simulink model "Ex3EMT"  (R2023b)
settings: Solver=VariableStepAuto  StartTime=0.0  StopTime=10.0  RelTol=1e-3
undefined symbols (not defined in the file): designMultirateFIR
libraries: dspmlti4 x8, dspstat3 x4
settings Model: Creator=Fartash  LastModifiedBy=Fartash

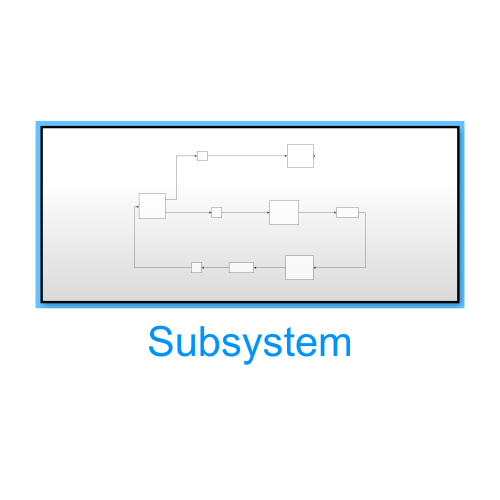
[thumbnail: Simulink's stored preview of the top-level diagram]
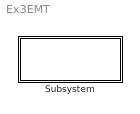
== system Ex3EMT ==
  Subsystem : Subsystem

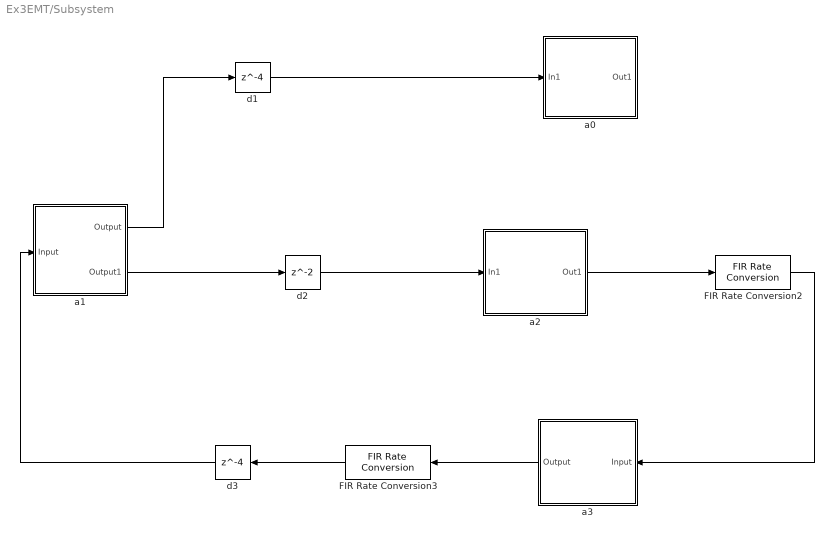
== system Ex3EMT/Subsystem ==
  FIR Rate Conversion2 : dspmlti4/FIR Rate Conversion  FilterSource=Auto  L=1  h=designMultirateFIR(3,2)  M=4  FilterObject=FRC  rateMode=Enforce single-rate processing  AllowArbitraryInputLength=off  roundingMode=Floor  overflowMode=off  firstCoeffDataTypeStr=Inherit: Same word length as input  firstCoeffMin=[]  firstCoeffMax=[]  firstCoeffLastDataTypeStr=Inherit: Same word length as input  outputDataTypeStr=Inherit: Same as accumulator  outputMin=[]  outputMax=[]  outputLastDataTypeStr=Inherit: Same as accumulator
  FIR Rate Conversion3 : dspmlti4/FIR Rate Conversion  FilterSource=Auto  L=3  h=designMultirateFIR(3,2)  M=1  FilterObject=FRC  rateMode=Enforce single-rate processing  AllowArbitraryInputLength=off  roundingMode=Floor  overflowMode=off  firstCoeffDataTypeStr=Inherit: Same word length as input  firstCoeffMin=[]  firstCoeffMax=[]  firstCoeffLastDataTypeStr=Inherit: Same word length as input  outputDataTypeStr=Inherit: Same as accumulator  outputMin=[]  outputMax=[]  outputLastDataTypeStr=Inherit: Same as accumulator
  a0 : Subsystem
  a1 : Subsystem
  a2 : Subsystem
  a3 : Subsystem
  d1 : Delay  DelayLength=4
  d2 : Delay
  d3 : Delay  DelayLength=4
  wires:
  FIR Rate Conversion3/1 -> d3/1
  a2/1(Out1) -> FIR Rate Conversion2/1
  a3/1(Output) -> FIR Rate Conversion3/1
  a1/1(Output) -> d1/1
  a1/2(Output1) -> d2/1
  d2/1 -> a2/1(In1)
  FIR Rate Conversion2/1 -> a3/1(Input)
  d1/1 -> a0/1(In1)
  d3/1 -> a1/1(Input)

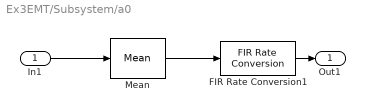
== system Ex3EMT/Subsystem/a0 ==
  In1 : Inport
  FIR Rate Conversion1 : dspmlti4/FIR Rate Conversion  FilterSource=Auto  L=3  h=designMultirateFIR(3,2)  M=1  FilterObject=FRC  rateMode=Enforce single-rate processing  AllowArbitraryInputLength=off  roundingMode=Floor  overflowMode=off  firstCoeffDataTypeStr=Inherit: Same word length as input  firstCoeffMin=[]  firstCoeffMax=[]  firstCoeffLastDataTypeStr=Inherit: Same word length as input  outputDataTypeStr=Inherit: Same as accumulator  outputMin=[]  outputMax=[]  outputLastDataTypeStr=Inherit: Same as accumulator
  Mean : dspstat3/Mean  run=off  InputProcessing=Columns as channels (frame based)  reset_popup=None  directionMode=Each column  dimension=1  roiEnable=off  roiType=Rectangles  roiPortion=Entire ROI  roiOutput=Individual statistics for each ROI  roiFlag=off  roundingMode=Floor  overflowMode=off  outputDataTypeStr=Inherit: Same as accumulator  outputMin=[]  outputMax=[]  outputLastDataTypeStr=Inherit: Same as accumulator
  Out1 : Outport
  wires:
  In1/1 -> Mean/1
  Mean/1 -> FIR Rate Conversion1/1
  FIR Rate Conversion1/1 -> Out1/1

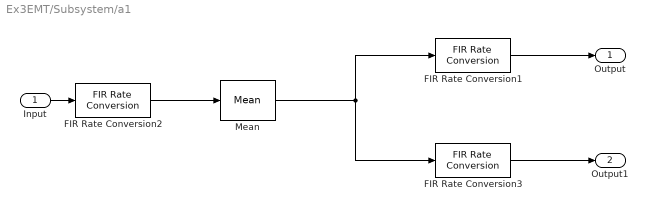
== system Ex3EMT/Subsystem/a1 ==
  Input : Inport
  FIR Rate Conversion1 : dspmlti4/FIR Rate Conversion  FilterSource=Auto  L=2  h=designMultirateFIR(3,2)  M=1  FilterObject=FRC  rateMode=Enforce single-rate processing  AllowArbitraryInputLength=off  roundingMode=Floor  overflowMode=off  firstCoeffDataTypeStr=Inherit: Same word length as input  firstCoeffMin=[]  firstCoeffMax=[]  firstCoeffLastDataTypeStr=Inherit: Same word length as input  outputDataTypeStr=Inherit: Same as accumulator  outputMin=[]  outputMax=[]  outputLastDataTypeStr=Inherit: Same as accumulator
  FIR Rate Conversion2 : dspmlti4/FIR Rate Conversion  FilterSource=Auto  L=4  h=designMultirateFIR(3,2)  M=1  FilterObject=FRC  rateMode=Enforce single-rate processing  AllowArbitraryInputLength=off  roundingMode=Floor  overflowMode=off  firstCoeffDataTypeStr=Inherit: Same word length as input  firstCoeffMin=[]  firstCoeffMax=[]  firstCoeffLastDataTypeStr=Inherit: Same word length as input  outputDataTypeStr=Inherit: Same as accumulator  outputMin=[]  outputMax=[]  outputLastDataTypeStr=Inherit: Same as accumulator
  FIR Rate Conversion3 : dspmlti4/FIR Rate Conversion  FilterSource=Auto  L=1  h=designMultirateFIR(3,2)  M=1  FilterObject=FRC  rateMode=Enforce single-rate processing  AllowArbitraryInputLength=off  roundingMode=Floor  overflowMode=off  firstCoeffDataTypeStr=Inherit: Same word length as input  firstCoeffMin=[]  firstCoeffMax=[]  firstCoeffLastDataTypeStr=Inherit: Same word length as input  outputDataTypeStr=Inherit: Same as accumulator  outputMin=[]  outputMax=[]  outputLastDataTypeStr=Inherit: Same as accumulator
  Mean : dspstat3/Mean  run=off  InputProcessing=Columns as channels (frame based)  reset_popup=None  directionMode=Each column  dimension=1  roiEnable=off  roiType=Rectangles  roiPortion=Entire ROI  roiOutput=Individual statistics for each ROI  roiFlag=off  roundingMode=Floor  overflowMode=off  outputDataTypeStr=Inherit: Same as accumulator  outputMin=[]  outputMax=[]  outputLastDataTypeStr=Inherit: Same as accumulator
  Output : Outport
  Output1 : Outport  Port=2
  wires:
  Input/1 -> FIR Rate Conversion2/1
  FIR Rate Conversion2/1 -> Mean/1
  FIR Rate Conversion3/1 -> Output1/1
  FIR Rate Conversion1/1 -> Output/1
  Mean/1 -> FIR Rate Conversion3/1, FIR Rate Conversion1/1

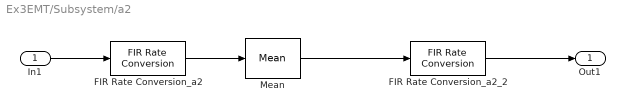
== system Ex3EMT/Subsystem/a2 ==
  In1 : Inport
  FIR Rate Conversion_a2 : dspmlti4/FIR Rate Conversion  FilterSource=Auto  L=3  h=designMultirateFIR(3,2)  M=1  FilterObject=FRC  rateMode=Enforce single-rate processing  AllowArbitraryInputLength=off  roundingMode=Floor  overflowMode=off  firstCoeffDataTypeStr=Inherit: Same word length as input  firstCoeffMin=[]  firstCoeffMax=[]  firstCoeffLastDataTypeStr=Inherit: Same word length as input  outputDataTypeStr=Inherit: Same as accumulator  outputMin=[]  outputMax=[]  outputLastDataTypeStr=Inherit: Same as accumulator
  FIR Rate Conversion_a2_2 : dspmlti4/FIR Rate Conversion  FilterSource=Auto  L=4  h=designMultirateFIR(3,2)  M=1  FilterObject=FRC  rateMode=Enforce single-rate processing  AllowArbitraryInputLength=off  roundingMode=Floor  overflowMode=off  firstCoeffDataTypeStr=Inherit: Same word length as input  firstCoeffMin=[]  firstCoeffMax=[]  firstCoeffLastDataTypeStr=Inherit: Same word length as input  outputDataTypeStr=Inherit: Same as accumulator  outputMin=[]  outputMax=[]  outputLastDataTypeStr=Inherit: Same as accumulator
  Mean : dspstat3/Mean  run=off  InputProcessing=Columns as channels (frame based)  reset_popup=None  directionMode=Each column  dimension=1  roiEnable=off  roiType=Rectangles  roiPortion=Entire ROI  roiOutput=Individual statistics for each ROI  roiFlag=off  roundingMode=Floor  overflowMode=off  outputDataTypeStr=Inherit: Same as accumulator  outputMin=[]  outputMax=[]  outputLastDataTypeStr=Inherit: Same as accumulator
  Out1 : Outport
  wires:
  Mean/1 -> FIR Rate Conversion_a2_2/1
  FIR Rate Conversion_a2_2/1 -> Out1/1
  In1/1 -> FIR Rate Conversion_a2/1
  FIR Rate Conversion_a2/1 -> Mean/1

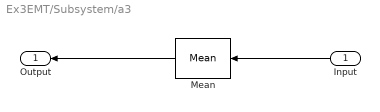
== system Ex3EMT/Subsystem/a3 ==
  Input : Inport
  Mean : dspstat3/Mean  run=off  InputProcessing=Columns as channels (frame based)  reset_popup=None  directionMode=Each column  dimension=1  roiEnable=off  roiType=Rectangles  roiPortion=Entire ROI  roiOutput=Individual statistics for each ROI  roiFlag=off  roundingMode=Floor  overflowMode=off  outputDataTypeStr=Inherit: Same as accumulator  outputMin=[]  outputMax=[]  outputLastDataTypeStr=Inherit: Same as accumulator
  Output : Outport
  wires:
  Mean/1 -> Output/1
  Input/1 -> Mean/1
